simulink model "case1_16AE10005"  (R2017b)
settings: Solver=ode4  StartTime=0.0  StopTime=10.0  FixedStep=0.0001  RelTol=1e-3
libraries: simulink x1
settings Model: Creator=ayushi  LastModifiedBy=ayushi

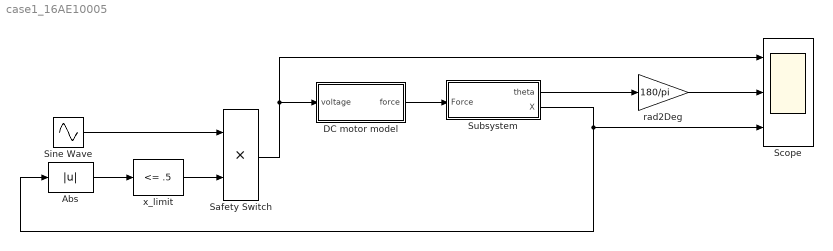
== system case1_16AE10005 ==
  Abs : Abs
  DC motor model : Subsystem
  Safety Switch : Product
  Scope : Scope  NumInputPorts=3
  Sine Wave : Sin  Amplitude=.3  Frequency=pi/2  SampleTime=0
  Subsystem : Subsystem
  rad2Deg : Gain  Gain=180/pi
  x_limit : simulink/Logic and Bit Operations/Compare To Constant  relop=<=  const=.5  OutDataTypeStr=boolean
  wires:
  DC motor model/1(force) -> Subsystem/1(Force)
  Subsystem/1("theta ") -> rad2Deg/1
  Safety Switch/1 -> Scope/1, DC motor model/1(voltage)
  Subsystem/2("X ") -> Abs/1, Scope/3
  Abs/1 -> x_limit/1
  Sine Wave/1 -> Safety Switch/1
  x_limit/1 -> Safety Switch/2
  rad2Deg/1 -> Scope/2

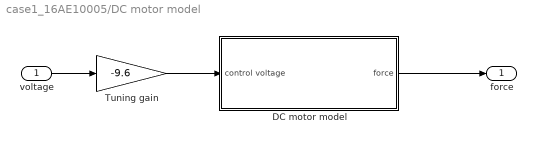
== system case1_16AE10005/DC motor model ==
  voltage : Inport
  DC motor model : Subsystem  mask{J=0.0000140, Kt=0.05, Kb=0.05, d=0.000001, R=2.5, L=0.0025}
      mask prompts: J "Moment of inertia"; Kt "Torque constant"; Kb "Electromotive force constant"; d "Linear approximation of viscous friction"; R "Electrical circuit resistance"; L "Electrical circuit inductance"
      mask Display: disp('DC motor')
  Tuning gain : Gain  Gain=-9.6
  force : Outport
  wires:
  Tuning gain/1 -> DC motor model/1(control voltage)
  voltage/1 -> Tuning gain/1
  DC motor model/1(force) -> force/1

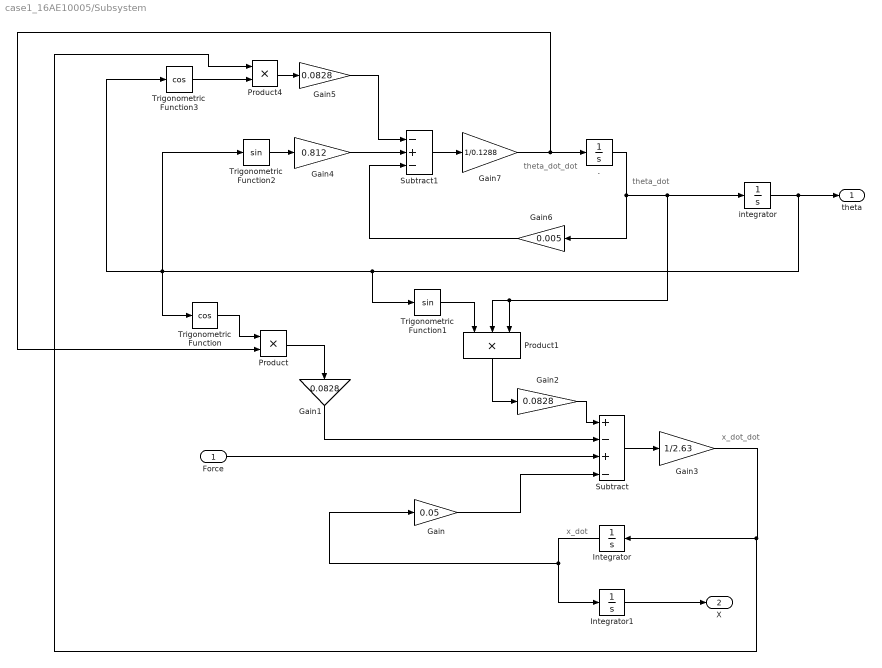
== system case1_16AE10005/Subsystem ==
  note: theta_dot
  note: theta_dot_dot
  note: x_dot
  note: x_dot_dot
  Force : Inport
  ". " : Integrator
  Gain : Gain  Gain=0.05
  Gain1 : Gain  Gain=0.0828
  Gain2 : Gain  Gain=0.0828
  Gain3 : Gain  Gain=1/2.63
  Gain4 : Gain  Gain=0.812
  Gain5 : Gain  Gain=0.0828
  Gain6 : Gain  Gain=0.005
  Gain7 : Gain  Gain=1/0.1288
  Integrator : Integrator
  Integrator1 : Integrator
  Product : Product
  Product1 : Product  Inputs=3
  Product4 : Product
  Subtract : Sum  Inputs=+-+-
  Subtract1 : Sum  Inputs=-+-
  Trigonometric Function : Trigonometry  Operator=cos
  Trigonometric Function1 : Trigonometry
  Trigonometric Function2 : Trigonometry
  Trigonometric Function3 : Trigonometry  Operator=cos
  integrator : Integrator
  "theta " : Outport
  "X " : Outport  Port=2
  wires:
  Trigonometric Function2/1 -> Gain4/1
  Integrator1/1 -> "X "/1
  integrator/1 -> "theta "/1, Trigonometric Function1/1, Trigonometric Function3/1, Trigonometric Function/1, Trigonometric Function2/1
  Gain/1 -> Subtract/4
  Integrator/1 -> Gain/1, Integrator1/1
  Gain3/1 -> Integrator/1, Product4/1
  Gain7/1 -> Product/2, ". "/1
  Product/1 -> Gain1/1
  Gain4/1 -> Subtract1/2
  Force/1 -> Subtract/3
  Product4/1 -> Gain5/1
  Trigonometric Function/1 -> Product/1
  Trigonometric Function1/1 -> Product1/1
  Trigonometric Function3/1 -> Product4/2
  Gain6/1 -> Subtract1/3
  ". "/1 -> Gain6/1, Product1/3, Product1/2, integrator/1
  Product1/1 -> Gain2/1
  Gain2/1 -> Subtract/1
  Gain1/1 -> Subtract/2
  Gain5/1 -> Subtract1/1
  Subtract/1 -> Gain3/1
  Subtract1/1 -> Gain7/1

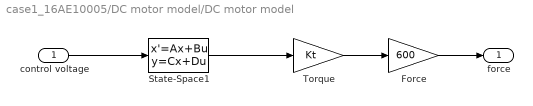
== system case1_16AE10005/DC motor model/DC motor model ==
  control voltage : Inport
  Force : Gain  Gain=600
  State-Space1 : StateSpace  A=[-d/J Kt/J;-Kb/L -R/L]  B=[0; 1/L]  C=[0 1]  D=0  InitialCondition=0
  Torque : Gain  Gain=Kt
  force : Outport
  wires:
  control voltage/1 -> State-Space1/1
  State-Space1/1 -> Torque/1
  Torque/1 -> Force/1
  Force/1 -> force/1
